simulink model "GridFormingConverter"  (R2025b)
settings: Solver=FixedStepAuto  StartTime=0.0  StopTime=simulationTime  FixedStep=gridInverter.vsm.samplingTime  MaxStep=gridInverter.vsm.samplingTime  RelTol=1e-3  AbsTol=1e-3
PreLoadFcn:
  | % Parameterize the model
  | GridFormingConverterInputParameters;
PostLoadFcn:
  | GridFormingConverterTestCondition;
undefined symbols (not defined in the file): base, DiscIntNeverNeededParam, Down, grid, gridInverter, k_smc1, k_smc2, L_smc, localSolverSampleTime, R_idsmc, scrFactorRg, scrFactorXg, transformer, TransmissionLine, Up
libraries: ee_lib x17, nesl_utility x17, eeGeneralControl x16, simulink x5, fl_lib x4, eeTransforms x4, eeSinGeneratorThreePhase x1, simulink_extras x1, eePowerMeasurement x1, eePwmGenerator x1
(part 2 of 3)

== system GridFormingConverter/Grid-Forming Converter/Grid-Forming Converter Control ==
  PrefPU : Inport
  QrefPU : Inport  Port=2
  IgabcPU : Inport  Port=3
  VgabcPU : Inport  Port=4
  Current Limiting : Subsystem
  Grid Voltage Reactive Power Support : Subsystem
  Measurement : Subsystem
      mask Display: image('$imagefile'); % Use "Edit Image" on toolstrip to change.
  Power Control : Subsystem
  Rate Transition3 : RateTransition
  VoltageCurrentControl : Subsystem
      settings: PortSchema="{\"entries\":[{\"content\":{\"sides\":[{\"content\":{\"connectorIds\":[\"In1\",\"In2\"]},\"type\":\"ConnectorPlacement.EquallySpacedRectSide\",\"uuid\":\"0bf15a12-7bc0-47e4-89bd-435769673763\"},{\"content\":{\"connectorIds\":[\"Out1\"],\"side\":\"RIGHT\"},\"type\":\"ConnectorPlacement.EquallySpacedRectSide\",\"uuid\":\"44a15d74-8878-4ec6-abe4-be0b1b609519\"},{\"content\":{\"connectorIds\":[\"In3\"],\"side\":\"TOP\"},\"type\":\"ConnectorPlacement.EquallySpacedRectSide\",\"uuid\":\"7a96781e-5638-4b2a-8101-d5785aae9f0f\"}]},\"type\":\"ConnectorPlacement.EquallySpacedConnector\",\"uuid\":\"4b3373ad-cf20-4175-894e-3bd1604dd0ce\"}],\"packageUris\":[\"http://schema.mathworks.com/mf0/Connector/R2020b\"],\"version\":\"1.0\"}"
  PmeasPU : Outport
  QmeasPU : Outport  Port=2
  FmeasHz : Outport  Port=3
  mabc : Outport  Port=4
  wires:
  VoltageCurrentControl/1(mabc) -> mabc/1
  VgabcPU/1 -> Measurement/1(Vgabcc)
  IgabcPU/1 -> Measurement/2(Igabc)
  Measurement/2(PmeasPU) -> PmeasPU/1
  Measurement/3(QmeasPU) -> QmeasPU/1
  Measurement/1(measure) -> Rate Transition3/1
  Power Control/3(angle) -> Measurement/3(Angle)
  Power Control/1(reactiveControl) -> Current Limiting/2(reactiveControl)
  Current Limiting/1(currentLimiting) -> VoltageCurrentControl/1(currentLimiting)
  QrefPU/1 -> Grid Voltage Reactive Power Support/3(QrefInput)
  PrefPU/1 -> Grid Voltage Reactive Power Support/2(PrefInput)
  Grid Voltage Reactive Power Support/1(Pref) -> Power Control/2(Pref)
  Grid Voltage Reactive Power Support/2(Qref) -> Power Control/3(Qref)
  Measurement/4(FmeasHz) -> FmeasHz/1
  Rate Transition3/1 -> Current Limiting/1(measure), VoltageCurrentControl/3(measure), Power Control/1(measure), Grid Voltage Reactive Power Support/1(measure)
  Power Control/2(activeControl) -> VoltageCurrentControl/2(activeControl)

== system GridFormingConverter/Grid-Forming Converter/Grid-Forming Converter Power Circuit ==
  mabc : Inport
  Average-Value : Subsystem  VariantControl=Average
  Switching : Subsystem  VariantControl=Switching
  P : PMIOPort  Side=Left
  N : PMIOPort  Port=2  Side=Left
  ABC : PMIOPort  Port=3  Side=Right

== system GridFormingConverter/Grid-Forming Converter/Grid-Forming Converter Control/Current Limiting ==
  In Bus Element : Inport  PortName=measure  Element=Igd
  In Bus Element1 : Inport  PortName=measure  Element=Igq
  In Bus Element2 : Inport  Port=2  PortName=reactiveControl  Element=Vmd
  In Bus Element4 : Inport  Port=2  PortName=reactiveControl  Element=Vmq
  CurrentLimitingMethod : Subsystem  Variant=on  VariantControlMode=label  VariantControl=Choice  LabelModeActiveChoice=virimp
  Subtract : Sum  Inputs=+-
  Subtract1 : Sum  Inputs=-+
  Out Bus Element : Outport  PortName=currentLimiting  Element=Vmd
  Out Bus Element1 : Outport  PortName=currentLimiting  Element=Vmq
  Out Bus Element2 : Outport  PortName=currentLimiting  Element=Idmax
  Out Bus Element3 : Outport  PortName=currentLimiting  Element=Iqmax
  wires:
  In Bus Element2/1 -> Subtract/1
  In Bus Element1/1 -> CurrentLimitingMethod/2(Igq)
  In Bus Element4/1 -> Subtract1/2
  Subtract/1 -> Out Bus Element/1
  Subtract1/1 -> Out Bus Element1/1
  In Bus Element/1 -> CurrentLimitingMethod/1(Igd)  "Q"
  CurrentLimitingMethod/1(delVd) -> Subtract/2
  CurrentLimitingMethod/2(delVq) -> Subtract1/1
  CurrentLimitingMethod/3(Idmax) -> Out Bus Element2/1
  CurrentLimitingMethod/4(Iqmax) -> Out Bus Element3/1

== system GridFormingConverter/Grid-Forming Converter/Grid-Forming Converter Control/Grid Voltage Reactive Power Support ==
  In Bus Element1 : Inport  PortName=measure  Element=Vgd
  In Bus Element3 : Inport  PortName=measure  Element=Vgq
  In Bus Element2 : Inport  PortName=measure  Element=Igd
  In Bus Element4 : Inport  PortName=measure  Element=Igq
  PrefInput : Inport  Port=2
  QrefInput : Inport  Port=3
  Modifying Active Power Reference : Subsystem
  Modifying Reactive Power Reference : Subsystem
  Rate Transition{,1..5} (6 alike) : RateTransition
  Pref : Outport
  Qref : Outport  Port=2
  wires:
  PrefInput/1 -> Modifying Active Power Reference/1(PrefInput)
  In Bus Element2/1 -> Modifying Active Power Reference/3(Igd)
  In Bus Element4/1 -> Modifying Active Power Reference/4(Igq)
  In Bus Element3/1 -> Rate Transition2/1
  QrefInput/1 -> Rate Transition3/1
  Modifying Reactive Power Reference/1(PrefNew) -> Rate Transition4/1
  Modifying Reactive Power Reference/2(QrefNew) -> Rate Transition5/1
  In Bus Element1/1 -> Rate Transition/1
  Modifying Active Power Reference/1(Pref) -> Rate Transition1/1
  Rate Transition2/1 -> Modifying Reactive Power Reference/2(Vgq)
  Rate Transition3/1 -> Modifying Reactive Power Reference/3(Qref)
  Rate Transition1/1 -> Modifying Reactive Power Reference/4(Pref)
  Rate Transition4/1 -> Pref/1
  Rate Transition5/1 -> Qref/1
  Rate Transition/1 -> Modifying Reactive Power Reference/1(Vgd), Modifying Active Power Reference/2(Vd)

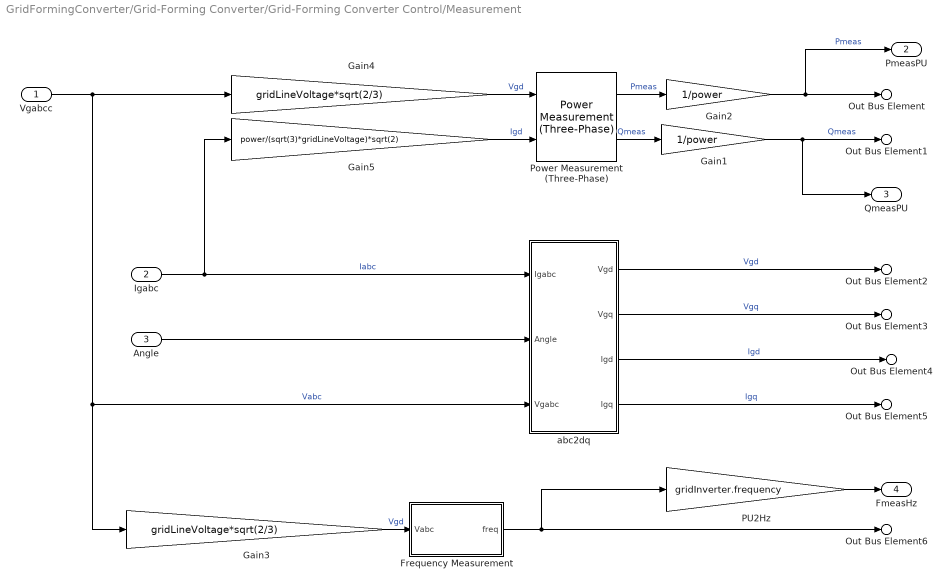
== system GridFormingConverter/Grid-Forming Converter/Grid-Forming Converter Control/Measurement ==
  Vgabcc : Inport
  Igabc : Inport  Port=2
  Angle : Inport  Port=3
  Frequency Measurement : Subsystem
  Gain1 : Gain  Gain=1/power
  Gain2 : Gain  Gain=1/power
  Gain3 : Gain  Gain=gridLineVoltage*sqrt(2/3)
  Gain4 : Gain  Gain=gridLineVoltage*sqrt(2/3)
  Gain5 : Gain  Gain=power/(sqrt(3)*gridLineVoltage)*sqrt(2)
  PU2Hz : Gain  Gain=gridInverter.frequency
  Power Measurement (Three-Phase) : eePowerMeasurement/Power Measurement (Three-Phase)  LabelModeActiveChoice=Discrete  F=powerFreq  K=[1]  Seq=Positive  Ts=measSampleTime
  abc2dq : Subsystem
  Out Bus Element : Outport  PortName=measure  Element=P
  Out Bus Element1 : Outport  PortName=measure  Element=Q
  Out Bus Element2 : Outport  PortName=measure  Element=Vgd
  Out Bus Element3 : Outport  PortName=measure  Element=Vgq
  Out Bus Element4 : Outport  PortName=measure  Element=Igd
  Out Bus Element5 : Outport  PortName=measure  Element=Igq
  Out Bus Element6 : Outport  PortName=measure  Element=fgrid
  PmeasPU : Outport  Port=2
  QmeasPU : Outport  Port=3
  FmeasHz : Outport  Port=4
  wires:
  Vgabcc/1 -> abc2dq/3(Vgabc), Gain3/1, Gain4/1  "Vabc"
  Angle/1 -> abc2dq/2(Angle)
  Igabc/1 -> Gain5/1, abc2dq/1(Igabc)  "Iabc"
  abc2dq/2(Vgq) -> Out Bus Element3/1  "Vgq"
  abc2dq/1(Vgd) -> Out Bus Element2/1  "Vgd"
  abc2dq/3(Igd) -> Out Bus Element4/1  "Igd"
  abc2dq/4(Igq) -> Out Bus Element5/1  "Igq"
  Frequency Measurement/1(freq) -> PU2Hz/1, Out Bus Element6/1
  PU2Hz/1 -> FmeasHz/1
  Power Measurement (Three-Phase)/1 -> Gain2/1  "Pmeas"
  Power Measurement (Three-Phase)/2 -> Gain1/1  "Qmeas"
  Gain4/1 -> Power Measurement (Three-Phase)/1  "Vgd"
  Gain5/1 -> Power Measurement (Three-Phase)/2  "Igd"
  Gain2/1 -> Out Bus Element/1, PmeasPU/1  "Pmeas"
  Gain1/1 -> QmeasPU/1, Out Bus Element1/1  "Qmeas"
  Gain3/1 -> Frequency Measurement/1(Vabc)  "Vgd"

== system GridFormingConverter/Grid-Forming Converter/Grid-Forming Converter Control/Power Control ==
  note: Reactive Power Control
  note: Active Power Control
  In Bus Element2 : Inport  PortName=measure  Element=P
  In Bus Element3 : Inport  PortName=measure  Element=Q
  In Bus Element1 : Inport  PortName=measure  Element=fgrid
  Pref : Inport  Port=2
  Qref : Inport  Port=3
  ActivePowerControl : Subsystem  Variant=on  VariantControlMode=label  VariantControl=Choice  LabelModeActiveChoice=vsm
  ReactiveControl : Subsystem
  Out Bus Element : Outport  PortName=reactiveControl  Element=Vmd
  Out Bus Element1 : Outport  PortName=reactiveControl  Element=Vmq
  Out Bus Element6 : Outport  Port=2  PortName=activeControl  Element=angle
  Out Bus Element4 : Outport  Port=2  PortName=activeControl  Element=w
  angle : Outport  Port=3
  wires:
  ActivePowerControl/2(w) -> Out Bus Element4/1
  In Bus Element3/1 -> ReactiveControl/2(Qmeas)
  ActivePowerControl/1(Theta) -> angle/1, Out Bus Element6/1
  ReactiveControl/1(Vmd) -> Out Bus Element/1
  ReactiveControl/2(Vmq) -> Out Bus Element1/1
  Pref/1 -> ActivePowerControl/1(Pref)  "Q"
  Qref/1 -> ReactiveControl/1(Qref)  "Q"
  In Bus Element2/1 -> ActivePowerControl/2(Pmeas)
  In Bus Element1/1 -> ActivePowerControl/3(fgrid)

== system GridFormingConverter/Grid-Forming Converter/Grid-Forming Converter Control/VoltageCurrentControl ==
  In Bus Element : Inport  PortName=currentLimiting  Element=Vmd
  In Bus Element1 : Inport  PortName=currentLimiting  Element=Vmq
  In Bus Element6 : Inport  PortName=currentLimiting  Element=Idmax
  In Bus Element7 : Inport  PortName=currentLimiting  Element=Iqmax
  Bus Element In6 : Inport  Port=2  PortName=activeControl  Element=w
  Bus Element In1 : Inport  Port=2  PortName=activeControl  Element=angle
  In Bus Element2 : Inport  Port=3  PortName=measure  Element=Vgd
  In Bus Element3 : Inport  Port=3  PortName=measure  Element=Vgq
  In Bus Element4 : Inport  Port=3  PortName=measure  Element=Igd
  In Bus Element5 : Inport  Port=3  PortName=measure  Element=Igq
  Controller : Subsystem
  Modulation Signal : Subsystem
  mabc : Outport
  wires:
  Controller/2(Vq) -> Modulation Signal/2(Vq)
  Modulation Signal/1(mabc) -> mabc/1
  Controller/1(Vd) -> Modulation Signal/1(Vd)
  In Bus Element4/1 -> Controller/6(Id)
  In Bus Element5/1 -> Controller/7(Iq)
  In Bus Element6/1 -> Controller/8(Idmax)
  In Bus Element7/1 -> Controller/9(Iqmax)
  In Bus Element2/1 -> Controller/4(Vsd)
  In Bus Element3/1 -> Controller/5(Vsq)
  Bus Element In6/1 -> Controller/1(Angfreq)
  In Bus Element/1 -> Controller/2(Vgdref)
  In Bus Element1/1 -> Controller/3(Vgqref)
  Bus Element In1/1 -> Modulation Signal/3(Angle)

== system GridFormingConverter/Grid-Forming Converter/Grid-Forming Converter Power Circuit/Average-Value ==
  mabc : Inport
  Electrical Reference : fl_lib/Electrical/Electrical Elements/Electrical Reference
  Grid Forming Converter : ee_lib/Semiconductors & Converters/Converters/Average-Value Voltage Source Converter (Three-Phase)  port_option=ee.enum.threePhasePort.composite  frequency_option=ee.enum.converters.frequency.variable  input_option=ee.enum.converters.inputOption.ModWave  FRated=50 Hz  losses_parameterization=ee.enum.converters.losses.fixed  Pfixed=10 W  ks=0.01  kc1=1.7 V  kc2=0.01 Ohm  Ploss_vect=[100, 800, 1870, 3250, 4900] W  Irms_vect=[10, 100, 200, 300, 400] A  Vdc_nom=300 V  thermal_mass=30000 J/K  temperature_specify=off  temperature_priority=High  temperature=298.15 K  temperature_nominal_specify=off  temperature_nominal_value=1  temperature_nominal_unit=K
      settings: InternalSimscapePortConfiguration="{\"Bottom\":[],\"Left\":[{\"id\":\"ModWave\",\"label\":\"ModWave\",\"type\":\"input\"},{\"id\":\"N\",\"label\":\"~\",\"type\":\"foundation.electrical.three_phase\"}],\"Right\":[{\"id\":\"p\",\"label\":\"+\",\"type\":\"foundation.electrical.electrical\"},{\"id\":\"n\",\"label\":\"-\",\"type\":\"foundation.electrical.electrical\"}],\"Top\":[]}"
  Simulink-PS Converter : nesl_utility/Simulink-PS Converter  PhysicalDomain=network_engine_domain  SubClassName=ps_input  LeftPortType=input  RightPortType=output  PseudoPeriodic=off  Frequencies=[]  NoiseDistribution=none  NoiseParameters=[]  Unit=1  AffineConversion=off  FilteringAndDerivatives=provide  SimscapeFilterOrder=1  InputFilterTimeConstant=0.001  UdotUserProvided=0
  P : PMIOPort  Side=Left
  N : PMIOPort  Port=2  Side=Left
  ABC : PMIOPort  Port=3  Side=Right
  wires:
  mabc/1 -> Simulink-PS Converter/1
  connections:
  ABC/RConn1 -- Grid Forming Converter/LConn2
  Simulink-PS Converter/RConn1 -- Grid Forming Converter/LConn1
  P/RConn1 -- Grid Forming Converter/RConn1
  Grid Forming Converter/RConn2 -- Electrical Reference/LConn1 -- N/RConn1

== system GridFormingConverter/Grid-Forming Converter/Grid-Forming Converter Power Circuit/Switching ==
  mabc : Inport
  Converter (Three-Phase) : ee_lib/Semiconductors & Converters/Converters/Converter (Three-Phase)  port_option=ee.enum.threePhasePort.composite  fidelity_option=ee.enum.converters.fidelity.detailed  device_type=ee.enum.converters.switchingdevice.ideal  showThermalPort=false  K=0  Vth=0.5 V  Vgt=1 V  Vgt_off=-1 V  Ih=1 A  Vf=0.8 V  Ron=0.001 Ohm  Rds=0.001 Ohm  Goff=1e-6 1/Ohm  Eon_scalar=22.86e-3 J  Eoff_scalar=17.14e-3 J  Eoff_natural_commutation=10e-3 J  Voff=300 V  Iout_scalar=600 A  onCurrentMeasDelay=0 s  useCurrentFromPreviousCycle=false  useVoltageFromPreviousCycle=false  diode_param=ee.enum.converters.protectiondiode.nodynamics  diode_Vf=0.01 V  diode_Ron=0.0001 Ohm  diode_Goff=1e-5 1/Ohm  diode_C=50 nF  diode_iRM=-235 A  diode_iF=300 A  diode_idot=-50 A/us  diode_trr_param=ee.enum.converters.diodetrr.trr_factor  diode_trr_factor=3  diode_trr=15 us  diode_Qrr=1500 s*uA  diode_rec_loss_model=ee.enum.diode.reverseRecoveryModel.fixed  diode_ErecVal=0 J  diode_scaleWithIandV=false  diode_ErecMat=zeros(2, 3) J  diode_TjrecVec=[298.15, 398.15] K  diode_IfrecVec=[.1, 1, 10] A  diode_IrecVal=10 A  diode_VrecVal=10 V  diode_tFilter=1 / 1000 / 100 s  thermal_network_parameterization=ee.enum.thermalNetworkTopology.external  Rth=[.08, .5] K/W  Rth_Cauer=[.08, .1, .5] K/W  Rth_Foster=[.08, .14, .22, .16] K/W  thermal_mass_parameterization=ee.enum.thermalNetwork.timeconstant  thermal_mass=[.01, .5] J/K  thermal_mass_Cauer=[.01, .1, .5] J/K  thermal_mass_Foster=[.001, .005, .05, .5] J/K  thermal_time_constant=[.001, .2] s  thermal_time_constant_Cauer=[.001, .1, .2] s  thermal_time_constant_Foster=[7e-05, .0007, .01, .08] s  thermal_mass_initial_temperatures=[25, 25] degC  thermal_mass_initial_temperatures_Cauer=[25, 25, 25] degC  junction_thermal_mass=0.01 J/K  Tvec_initial_Foster=[25, 25, 25, 25] degC  snubber_type=ee.enum.converters.snubber.exclude  Cs=1e-7 F  Rs=0.1 Ohm  Vce_loss=[0, 150, 300] V
  Mod2PWM SIgnal : Subsystem
  Simulink-PS Converter{1..6} (6 alike) : nesl_utility/Simulink-PS Converter  PhysicalDomain=network_engine_domain  SubClassName=ps_input  LeftPortType=input  RightPortType=output  PseudoPeriodic=off  Frequencies=[]  NoiseDistribution=none  NoiseParameters=[]  Unit=1  AffineConversion=off  FilteringAndDerivatives=provide  SimscapeFilterOrder=1  InputFilterTimeConstant=0.001  UdotUserProvided=0
  Six-Pulse Gate Multiplexer : ee_lib/Semiconductors & Converters/Converters/Six-Pulse Gate Multiplexer  port_option=ee.enum.controlport.ps
  P : PMIOPort  Side=Left
  N : PMIOPort  Port=2  Side=Left
  ABC : PMIOPort  Port=3  Side=Right
  wires:
  mabc/1 -> Mod2PWM SIgnal/1(mod)
  Mod2PWM SIgnal/1(AH) -> Simulink-PS Converter6/1
  Mod2PWM SIgnal/2(AL) -> Simulink-PS Converter5/1
  Mod2PWM SIgnal/3(BH) -> Simulink-PS Converter4/1
  Mod2PWM SIgnal/4(BL) -> Simulink-PS Converter3/1
  Mod2PWM SIgnal/5(CH) -> Simulink-PS Converter2/1
  Mod2PWM SIgnal/6(CL) -> Simulink-PS Converter1/1
  connections:
  Six-Pulse Gate Multiplexer/RConn1 -- Converter (Three-Phase)/LConn1
  P/RConn1 -- Converter (Three-Phase)/RConn1
  Six-Pulse Gate Multiplexer/LConn2 -- Simulink-PS Converter5/RConn1
  Simulink-PS Converter2/RConn1 -- Six-Pulse Gate Multiplexer/LConn5
  Simulink-PS Converter1/RConn1 -- Six-Pulse Gate Multiplexer/LConn6
  Six-Pulse Gate Multiplexer/LConn1 -- Simulink-PS Converter6/RConn1
  N/RConn1 -- Converter (Three-Phase)/RConn2
  Six-Pulse Gate Multiplexer/LConn3 -- Simulink-PS Converter4/RConn1
  Six-Pulse Gate Multiplexer/LConn4 -- Simulink-PS Converter3/RConn1
  Converter (Three-Phase)/LConn2 -- ABC/RConn1

== system GridFormingConverter/Grid-Forming Converter/Grid-Forming Converter Control/Current Limiting/CurrentLimitingMethod ==
  Igd : Inport
  Igq : Inport  Port=2
  currentLimitAndVirtual : Subsystem  VariantControl=both
  currentSaturation : Subsystem  VariantControl=ctSat
  virtualImpedance : Subsystem  VariantControl=virimp
  delVd : Outport
  delVq : Outport  Port=2
  Idmax : Outport  Port=3
  Iqmax : Outport  Port=4

== system GridFormingConverter/Grid-Forming Converter/Grid-Forming Converter Control/Grid Voltage Reactive Power Support/Modifying Active Power Reference ==
  PrefInput : Inport
  Vd : Inport  Port=2
  Igd : Inport  Port=3
  Igq : Inport  Port=4
  AND : Logic  IconShape=distinctive  AllPortsSameDT=off  OutDataTypeStr=boolean
  Abs : Abs  SaturateOnIntegerOverflow=off
  Compare To Constant : simulink/Logic and Bit Operations/Compare To Constant  relop=<=  const=0.90  OutDataTypeStr=boolean
  Computing New Active Power Ref : Subsystem
  Math Function1 : Math  Operator=hypot
  Power Sign : Signum
  Product : Product
  Rate Transition1 : RateTransition
  Relay : Relay  OnSwitchValue=maxVICurrentLimit*0.96  OffSwitchValue=1
  Switch : Switch  Criteria=u2 > Threshold  SaturateOnIntegerOverflow=off  InputSameDT=off
  Pref : Outport
  wires:
  Computing New Active Power Ref/1(Pref) -> Switch/1
  Math Function1/1 -> Rate Transition1/1  "Is"
  Vd/1 -> Computing New Active Power Ref/2(Vd), Compare To Constant/1
  PrefInput/1 -> Power Sign/1, Switch/3
  Igd/1 -> Math Function1/2
  Switch/1 -> Abs/1
  Abs/1 -> Product/1
  Power Sign/1 -> Product/2
  Product/1 -> Pref/1
  Relay/1 -> AND/2
  AND/1 -> Switch/2
  Compare To Constant/1 -> AND/1
  Igq/1 -> Computing New Active Power Ref/1(Iq), Math Function1/1
  Rate Transition1/1 -> Relay/1

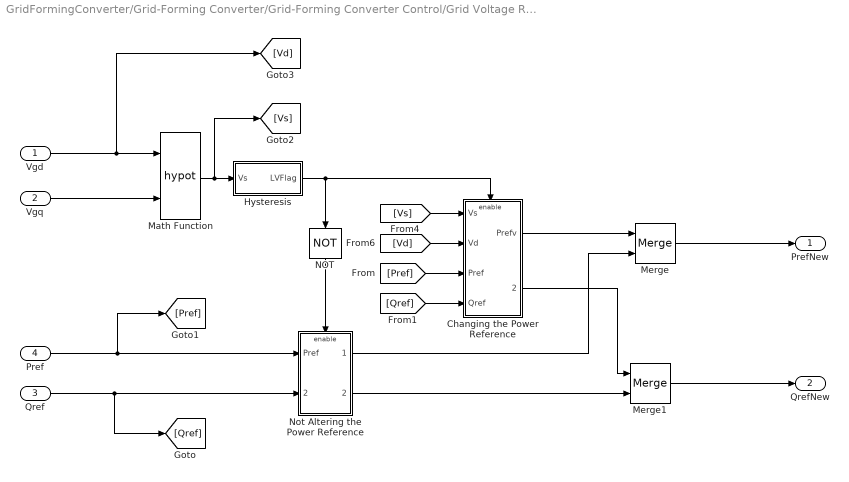
== system GridFormingConverter/Grid-Forming Converter/Grid-Forming Converter Control/Grid Voltage Reactive Power Support/Modifying Reactive Power Reference ==
  Vgd : Inport
  Vgq : Inport  Port=2
  Qref : Inport  Port=3
  Pref : Inport  Port=4
  Changing the Power Reference : Subsystem
  Hysteresis : Subsystem
  Math Function : Math  Operator=hypot
  Merge : Merge
  Merge1 : Merge
  NOT : Logic  Operator=NOT  IconShape=distinctive  AllPortsSameDT=off  OutDataTypeStr=boolean
  Not Altering the Power Reference : Subsystem
  PrefNew : Outport
  QrefNew : Outport  Port=2
  wires:
  Vgd/1 -> [Vd], Math Function/1
  Not Altering the Power Reference/2(Qrefv) -> Merge1/2
  Math Function/1 -> Hysteresis/1(Vs), [Vs]
  [Vs] -> Changing the Power Reference/1(Vs)
  Not Altering the Power Reference/1(Prefv) -> Merge/2
  Changing the Power Reference/1(Prefv) -> Merge/1
  NOT/1 -> Not Altering the Power Reference/Enable
  Qref/1 -> Not Altering the Power Reference/2(Qref), [Qref]
  Hysteresis/1(LVFlag) -> Changing the Power Reference/Enable, NOT/1
  [Vd] -> Changing the Power Reference/2(Vd)
  Changing the Power Reference/2(Qrefv) -> Merge1/1
  Vgq/1 -> Math Function/2
  Pref/1 -> Not Altering the Power Reference/1(Pref), [Pref]
  Merge1/1 -> QrefNew/1
  Merge/1 -> PrefNew/1
  [Pref] -> Changing the Power Reference/3(Pref)
  [Qref] -> Changing the Power Reference/4(Qref)

== system GridFormingConverter/Grid-Forming Converter/Grid-Forming Converter Control/Measurement/Frequency Measurement ==
  Vabc : Inport
  Convert To PU : Gain  Gain=1/powerFreq
  Frequency Measurement : Subsystem  TreatAsAtomicUnit=on  SystemSampleTime=sampleTime  mask{initialFrequency=powerFreq, sampleTime=activePowerSampleTime}
      mask prompts: initialFrequency "Initial frequency in Hz"; sampleTime "Sample time in sec"
      mask DialogControl Container7 Prompt: General
  Low-Pass Filter : eeGeneralControl/Low-Pass Filter (Discrete or Continuous)  K=1  T=freqMeasTimeConst  B=inf  A=-inf  init_option=Inherited from block input  x0=0  Ts=-1
  Low-Pass Filter1 : eeGeneralControl/Low-Pass Filter (Discrete or Continuous)  K=1  T=0.1/powerFreq  B=inf  A=-inf  init_option=Inherited from block input  x0=0  Ts=-1
  Saturation : Saturate  UpperLimit=1.1  LowerLimit=0.9
  freq : Outport
  wires:
  Low-Pass Filter/1 -> Convert To PU/1  "Freq"
  Frequency Measurement/1(Freq) -> Low-Pass Filter/1
  Convert To PU/1 -> Saturation/1
  Vabc/1 -> Low-Pass Filter1/1
  Low-Pass Filter1/1 -> Frequency Measurement/1(abc)
  Saturation/1 -> freq/1

== system GridFormingConverter/Grid-Forming Converter/Grid-Forming Converter Control/Measurement/abc2dq ==
  Igabc : Inport
  Angle : Inport  Port=2
  Vgabc : Inport  Port=3
  Supply Current to dq : Subsystem
  Supply Voltage  to dq : Subsystem
  Vgd : Outport
  Vgq : Outport  Port=2
  Igd : Outport  Port=3
  Igq : Outport  Port=4
  wires:
  Angle/1 -> Supply Voltage  to dq/1(Angle), Supply Current to dq/2(Angle)
  Vgabc/1 -> Supply Voltage  to dq/2(abc)
  Igabc/1 -> Supply Current to dq/1(abc)
  Supply Current to dq/1(Igd) -> Igd/1  "Id"
  Supply Current to dq/2(Igq) -> Igq/1  "Iq"
  Supply Voltage  to dq/1(Vgd) -> Vgd/1  "Vgd"
  Supply Voltage  to dq/2(Vgq) -> Vgq/1  "Vgq"

== system GridFormingConverter/Grid-Forming Converter/Grid-Forming Converter Control/Power Control/ActivePowerControl ==
  Pref : Inport
  Pmeas : Inport  Port=2
  fgrid : Inport  Port=3
  droopControl : Subsystem  VariantControl=droop
  vsmControl : Subsystem  VariantControl=vsm
  Theta : Outport
  w : Outport  Port=2

== system GridFormingConverter/Grid-Forming Converter/Grid-Forming Converter Control/Power Control/ReactiveControl ==
  note: Vs-delV
  Qref : Inport
  Qmeas : Inport  Port=2
  Constant : Constant  Value=voltreference
  Constant2 : Constant  Value=0
  Gain : Gain  Gain=QVoltDroop
  Low-Pass Filter (Discrete or Continuous) : eeGeneralControl/Low-Pass Filter (Discrete or Continuous)  K=1  T=QVoltFilterTC  B=inf  A=-inf  init_option=Specify as parameter  x0=0  Ts=activePowerSampleTime
  Product1 : Product
  Saturation1 : Saturate  UpperLimit=(dcBusVoltage/2)/(sqrt(2/3)*gridLineVoltage)  LowerLimit=-(dcBusVoltage/2)/(sqrt(2/3)*gridLineVoltage)
  Sum : Sum  Inputs=|+-
  Sum1 : Sum  Inputs=|++
  Vmd : Outport
  Vmq : Outport  Port=2
  wires:
  Sum/1 -> Gain/1
  Qmeas/1 -> Low-Pass Filter (Discrete or Continuous)/1
  Low-Pass Filter (Discrete or Continuous)/1 -> Sum/2
  Gain/1 -> Sum1/1
  Product1/1 -> Saturation1/1  "Q"
  Constant/1 -> Product1/2, Sum1/2
  Constant2/1 -> Vmq/1
  Sum1/1 -> Product1/1
  Qref/1 -> Sum/1
  Saturation1/1 -> Vmd/1

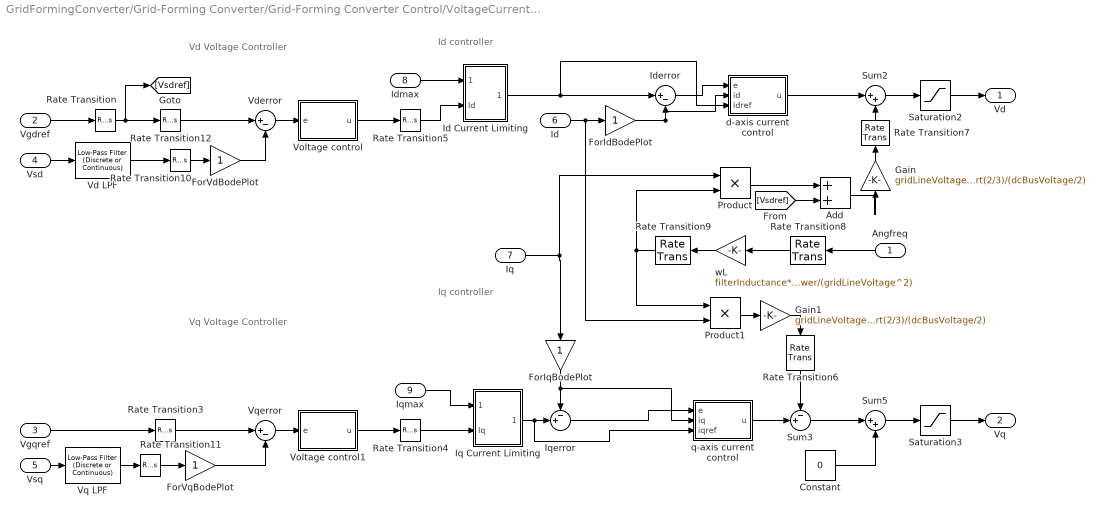
== system GridFormingConverter/Grid-Forming Converter/Grid-Forming Converter Control/VoltageCurrentControl/Controller ==
  note: Id controller
  note: Vd Voltage Controller
  note: Iq controller
  note: Vq Voltage Controller
  Angfreq : Inport
  Vgdref : Inport  Port=2
  Vgqref : Inport  Port=3
  Vsd : Inport  Port=4
  Vsq : Inport  Port=5
  Id : Inport  Port=6
  Iq : Inport  Port=7
  Idmax : Inport  Port=8
  Iqmax : Inport  Port=9
  Add : Sum
  Constant : Constant  Value=0  SampleTime=currentControlTs
  ForIdBodePlot : Gain
  ForIqBodePlot : Gain
  ForVdBodePlot : Gain
  ForVqBodePlot : Gain
  Gain : Gain  Gain=gridLineVoltage*sqrt(2/3)/(dcBusVoltage/2)
  Gain1 : Gain  Gain=gridLineVoltage*sqrt(2/3)/(dcBusVoltage/2)
  Id Current Limiting : Subsystem
  Iderror : Sum  Inputs=|+-
  Iq Current Limiting : Subsystem
  Iqerror : Sum  Inputs=-+|
  Product : Product
  Product1 : Product
  Rate Transition{,3..12} (11 alike) : RateTransition
  Saturation2 : Saturate  UpperLimit=4  LowerLimit=-3
  Saturation3 : Saturate  UpperLimit=3  LowerLimit=-3
  Sum2 : Sum  Inputs=|++
  Sum3 : Sum  Inputs=-+|
  Sum5 : Sum  Inputs=|++
  Vd LPF : eeGeneralControl/Low-Pass Filter (Discrete or Continuous)  K=1  T=vdvqLPFTimeConst  B=inf  A=-inf  init_option=Specify as parameter  x0=0  Ts=voltControlTs
  Vderror : Sum  Inputs=|+-
  Voltage control : Subsystem
  Voltage control1 : Subsystem
  Vq LPF : eeGeneralControl/Low-Pass Filter (Discrete or Continuous)  K=1  T=vdvqLPFTimeConst  B=inf  A=-inf  init_option=Inherited from block input  x0=0  Ts=voltControlTs
  Vqerror : Sum  Inputs=|+-
  d-axis current control : Subsystem
  q-axis current control : Subsystem
  wL : Gain  Gain=filterInductance*power/(gridLineVoltage^2)
  Vd : Outport  VectorParamsAs1DForOutWhenUnconnected=off
  Vq : Outport  Port=2  VectorParamsAs1DForOutWhenUnconnected=off
  wires:
  Iqerror/1 -> q-axis current control/1(e)
  wL/1 -> Rate Transition9/1
  Iq/1 -> ForIqBodePlot/1, Product/1
  Angfreq/1 -> Rate Transition8/1
  Constant/1 -> Sum5/2
  Iderror/1 -> d-axis current control/1(e)
  Saturation3/1 -> Vq/1
  Saturation2/1 -> Vd/1
  Product1/1 -> Gain1/1
  Product/1 -> Add/1
  d-axis current control/1(u) -> Sum2/1
  q-axis current control/1(u) -> Sum3/2
  Sum3/1 -> Sum5/1
  Vsq/1 -> Vq LPF/1
  Id/1 -> Product1/2, ForIdBodePlot/1
  Vderror/1 -> Voltage control/1(e)
  Iqmax/1 -> Iq Current Limiting/1(Imax)
  Vgqref/1 -> Rate Transition3/1
  Vqerror/1 -> Voltage control1/1(e)
  Gain1/1 -> Rate Transition6/1
  [Vsdref] -> Add/2
  Add/1 -> Gain/1
  Gain/1 -> Rate Transition7/1
  Voltage control/1(u) -> Rate Transition5/1
  Idmax/1 -> Id Current Limiting/1(Imax)
  Iq Current Limiting/1(Iqref) -> q-axis current control/3(iqref), Iqerror/2
  Voltage control1/1(u) -> Rate Transition4/1
  Vsd/1 -> Vd LPF/1
  ForIdBodePlot/1 -> d-axis current control/2(id), Iderror/2
  ForIqBodePlot/1 -> q-axis current control/2(iq), Iqerror/1
  Id Current Limiting/1(Idref) -> d-axis current control/3(idref), Iderror/1
  Vgdref/1 -> Rate Transition/1
  Rate Transition/1 -> [Vsdref], Rate Transition12/1
  Rate Transition3/1 -> Vqerror/1
  Rate Transition4/1 -> Iq Current Limiting/2(Iq)
  Rate Transition5/1 -> Id Current Limiting/2(Id)
  Rate Transition6/1 -> Sum3/1
  Rate Transition7/1 -> Sum2/2
  Rate Transition8/1 -> wL/1
  Vq LPF/1 -> Rate Transition11/1
  Rate Transition9/1 -> Product/2, Product1/1
  ForVdBodePlot/1 -> Vderror/2
  ForVqBodePlot/1 -> Vqerror/2
  Vd LPF/1 -> Rate Transition10/1
  Rate Transition10/1 -> ForVdBodePlot/1
  Rate Transition11/1 -> ForVqBodePlot/1
  Rate Transition12/1 -> Vderror/1
  Sum5/1 -> Saturation3/1
  Sum2/1 -> Saturation2/1

== system GridFormingConverter/Grid-Forming Converter/Grid-Forming Converter Control/VoltageCurrentControl/Modulation Signal ==
  Vd : Inport
  Vq : Inport  Port=2
  Angle : Inport  Port=3
  Constant : Constant  Value=0
  Inverse Park Transform : eeTransforms/Inverse Park Transform  AxisAlignment=D-axis  PowerInvariant=off
  Mux1 : Mux  Inputs=3
  Saturation2 : Saturate  UpperLimit=1  LowerLimit=-1
  mabc : Outport  VectorParamsAs1DForOutWhenUnconnected=off
  wires:
  Inverse Park Transform/1 -> Saturation2/1
  Mux1/1 -> Inverse Park Transform/1
  Saturation2/1 -> mabc/1
  Constant/1 -> Mux1/3
  Vd/1 -> Mux1/1
  Angle/1 -> Inverse Park Transform/2
  Vq/1 -> Mux1/2

== system GridFormingConverter/Grid-Forming Converter/Grid-Forming Converter Power Circuit/Switching/Mod2PWM SIgnal ==
  mod : Inport
  Add : Sum
  Constant : Constant
  Constant1 : Constant
  Demux : Demux  Outputs=3
  Demux1 : Demux  Outputs=3
  Gain : Gain
  Gain1 : Gain  Gain=0.5
  PWM Generator : eePwmGenerator/PWM Generator  CarrCount=Up-Down  Tper=1/gridInverter.switchingFrequency  Tdelay=0  Ts=1/(10*gridInverter.switchingFrequency)
  Rate Transition1 : RateTransition  OutPortSampleTime=1/(10*gridInverter.switchingFrequency)
  Subtract : Sum  Inputs=-+
  AH : Outport
  AL : Outport  Port=2
  BH : Outport  Port=3
  BL : Outport  Port=4
  CH : Outport  Port=5
  CL : Outport  Port=6
  wires:
  Gain/1 -> Demux/1, Subtract/1
  Gain1/1 -> Rate Transition1/1
  Constant1/1 -> Add/2
  PWM Generator/1 -> Gain/1
  mod/1 -> Add/1
  Add/1 -> Gain1/1
  Rate Transition1/1 -> PWM Generator/1
  Subtract/1 -> Demux1/1
  Constant/1 -> Subtract/2
  Demux1/2 -> BL/1
  Demux1/3 -> CL/1
  Demux/1 -> AH/1
  Demux1/1 -> AL/1
  Demux/2 -> BH/1
  Demux/3 -> CH/1

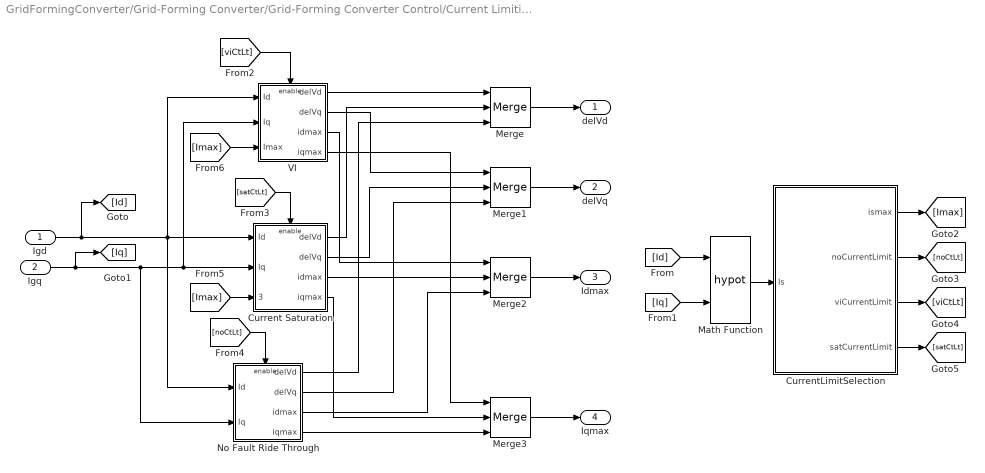
== system GridFormingConverter/Grid-Forming Converter/Grid-Forming Converter Control/Current Limiting/CurrentLimitingMethod/currentLimitAndVirtual ==
  Igd : Inport
  Igq : Inport  Port=2
  Current Saturation : Subsystem
  CurrentLimitSelection : Stateflow chart  TreatAsAtomicUnit=on
  Math Function : Math  Operator=hypot
  Merge{,1..3} (4 alike) : Merge  Inputs=3
  No Fault Ride Through : Subsystem
  VI : Subsystem
  delVd : Outport
  delVq : Outport  Port=2
  Idmax : Outport  Port=3
  Iqmax : Outport  Port=4
  wires:
  Merge2/1 -> Idmax/1
  Igq/1 -> Current Saturation/2(Iq), VI/2(Iq), No Fault Ride Through/2(Iq), [Iq]
  Merge1/1 -> delVq/1
  Igd/1 -> VI/1(Id), Current Saturation/1(Id), No Fault Ride Through/1(Id), [Id]
  No Fault Ride Through/1(delVd) -> Merge/3
  No Fault Ride Through/3(idmax) -> Merge2/3
  VI/1(delVd) -> Merge/1
  [Iq] -> Math Function/2
  [Id] -> Math Function/1
  Current Saturation/1(delVd) -> Merge/2
  Current Saturation/4(iqmax) -> Merge3/2
  Merge/1 -> delVd/1
  VI/2(delVq) -> Merge1/1
  Current Saturation/3(idmax) -> Merge2/2
  VI/4(iqmax) -> Merge3/1
  VI/3(idmax) -> Merge2/1
  No Fault Ride Through/4(iqmax) -> Merge3/3
  Current Saturation/2(delVq) -> Merge1/2
  Merge3/1 -> Iqmax/1
  No Fault Ride Through/2(delVq) -> Merge1/3
  Math Function/1 -> CurrentLimitSelection/1(Is)
  CurrentLimitSelection/1(ismax) -> [Imax]
  CurrentLimitSelection/2(noCurrentLimit) -> [noCtLt]
  CurrentLimitSelection/3(viCurrentLimit) -> [viCtLt]
  CurrentLimitSelection/4(satCurrentLimit) -> [satCtLt]
  [viCtLt] -> VI/Enable
  [satCtLt] -> Current Saturation/Enable
  [noCtLt] -> No Fault Ride Through/Enable
  [Imax] -> Current Saturation/3(Imaxsat)
  [Imax] -> VI/3(Imax)

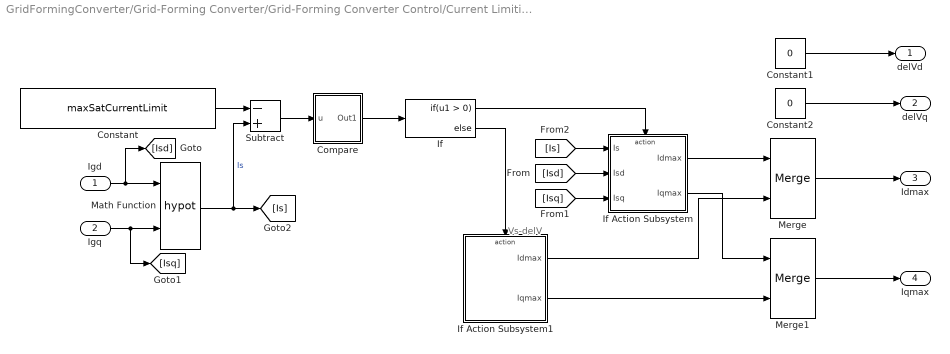
== system GridFormingConverter/Grid-Forming Converter/Grid-Forming Converter Control/Current Limiting/CurrentLimitingMethod/currentSaturation ==
  note: Vs-delV
  Igd : Inport
  Igq : Inport  Port=2
  Compare : Subsystem
  Constant : Constant  Value=maxSatCurrentLimit
  Constant1 : Constant  Value=0
  Constant2 : Constant  Value=0
  If : If
  If Action Subsystem : Subsystem  TreatAsAtomicUnit=on
  If Action Subsystem1 : Subsystem  TreatAsAtomicUnit=on
  Math Function : Math  Operator=hypot
  Merge : Merge
  Merge1 : Merge
  Subtract : Sum  Inputs=-+
  delVd : Outport
  delVq : Outport  Port=2
  Idmax : Outport  Port=3
  Iqmax : Outport  Port=4
  wires:
  Igd/1 -> [Isd], Math Function/1
  Igq/1 -> [Isq], Math Function/2
  Constant/1 -> Subtract/1
  Math Function/1 -> [Is], Subtract/2  "Is"
  If/1 -> If Action Subsystem/Action
  [Isd] -> If Action Subsystem/2(Isd)
  [Isq] -> If Action Subsystem/3(Isq)
  Subtract/1 -> Compare/1(u)
  Compare/1(Out1) -> If/1
  If/2 -> If Action Subsystem1/Action
  [Is] -> If Action Subsystem/1(Is)
  If Action Subsystem/1(Idmax) -> Merge/1
  If Action Subsystem1/1(Idmax) -> Merge/2
  If Action Subsystem/2(Iqmax) -> Merge1/1
  If Action Subsystem1/2(Iqmax) -> Merge1/2
  Constant2/1 -> delVq/1
  Constant1/1 -> delVd/1
  Merge/1 -> Idmax/1
  Merge1/1 -> Iqmax/1

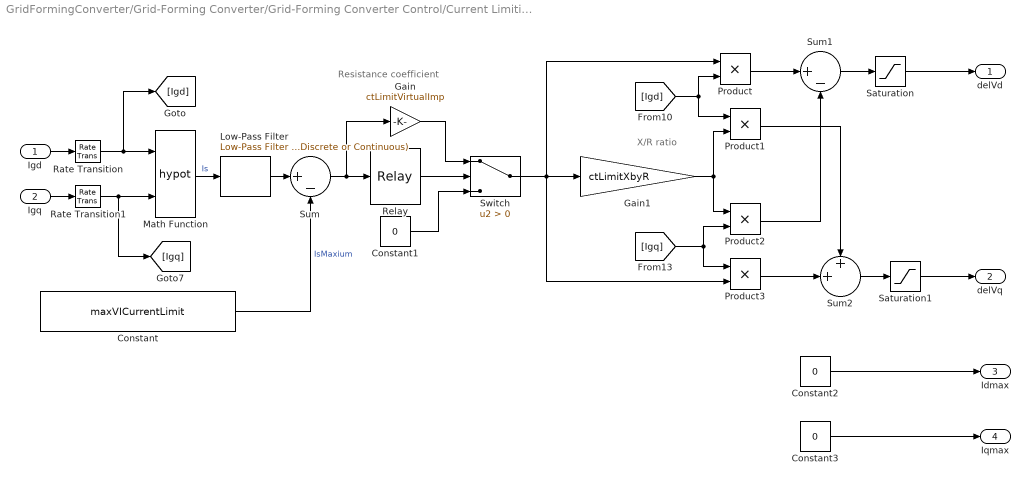
== system GridFormingConverter/Grid-Forming Converter/Grid-Forming Converter Control/Current Limiting/CurrentLimitingMethod/virtualImpedance ==
  note: X/R ratio
  note: Resistance coefficient
  Igd : Inport
  Igq : Inport  Port=2
  Constant : Constant  Value=maxVICurrentLimit
  Constant1 : Constant  Value=0
  Constant2 : Constant  Value=0
  Constant3 : Constant  Value=0
  Gain : Gain  Gain=ctLimitVirtualImp
  Gain1 : Gain  Gain=ctLimitXbyR
  Low-Pass Filter : eeGeneralControl/Low-Pass Filter (Discrete or Continuous)  K=1  T=currentVITimeConst  B=inf  A=-inf  init_option=Inherited from block input  x0=0  Ts=-1
  Math Function : Math  Operator=hypot
  Product{,1..3} (4 alike) : Product
  Rate Transition : RateTransition
  Rate Transition1 : RateTransition
  Relay : Relay  OnSwitchValue=0.01  OffSwitchValue=-0.05
  Saturation : Saturate  UpperLimit=1  LowerLimit=-1
  Saturation1 : Saturate  UpperLimit=1  LowerLimit=-1
  Sum : Sum  Inputs=|+-
  Sum1 : Sum  Inputs=|+-
  Sum2 : Sum  Inputs=++|
  Switch : Switch  Criteria=u2 > Threshold  SaturateOnIntegerOverflow=off  InputSameDT=off
  delVd : Outport
  delVq : Outport  Port=2
  Idmax : Outport  Port=3
  Iqmax : Outport  Port=4
  wires:
  Sum/1 -> Gain/1, Relay/1
  Igq/1 -> Rate Transition1/1
  Product1/1 -> Sum2/1
  Gain1/1 -> Product1/2, Product2/1
  Sum1/1 -> Saturation/1
  Product/1 -> Sum1/1
  Product2/1 -> Sum1/2
  Constant/1 -> Sum/2  "IsMaxium"
  Math Function/1 -> Low-Pass Filter/1  "Is"
  [Igq] -> Product3/1, Product2/2
  Switch/1 -> Gain1/1, Product3/2, Product/1
  [Igd] -> Product1/1, Product/2
  Constant2/1 -> Idmax/1
  Constant3/1 -> Iqmax/1
  Gain/1 -> Switch/1
  Constant1/1 -> Switch/3
  Igd/1 -> Rate Transition/1
  Saturation1/1 -> delVq/1
  Relay/1 -> Switch/2
  Saturation/1 -> delVd/1
  Low-Pass Filter/1 -> Sum/1
  Product3/1 -> Sum2/2
  Sum2/1 -> Saturation1/1
  Rate Transition/1 -> Math Function/1, [Igd]
  Rate Transition1/1 -> [Igq], Math Function/2

== system GridFormingConverter/Grid-Forming Converter/Grid-Forming Converter Control/Grid Voltage Reactive Power Support/Modifying Active Power Reference/Computing New Active Power Ref ==
  Iq : Inport
  Vd : Inport  Port=2
  Abs : Abs  SaturateOnIntegerOverflow=off
  Constant : Constant  Value=maxVICurrentLimit*0.96
  Constant1 : Constant  Value=0
  Product : Product
  Sqrt : Sqrt
  Square : Math  Operator=square
  Square1 : Math  Operator=square
  Subtract : Sum  Inputs=-+
  Switch : Switch  Criteria=u2 > Threshold  Threshold=1.15  SaturateOnIntegerOverflow=off  InputSameDT=off
  Pref : Outport
  wires:
  Constant/1 -> Square1/1
  Switch/1 -> Product/2
  Square/1 -> Subtract/1
  Square1/1 -> Subtract/2
  Vd/1 -> Product/1
  Sqrt/1 -> Abs/1
  Iq/1 -> Square/1
  Product/1 -> Pref/1
  Subtract/1 -> Switch/2, Sqrt/1
  Constant1/1 -> Switch/3
  Abs/1 -> Switch/1

== system GridFormingConverter/Grid-Forming Converter/Grid-Forming Converter Control/Grid Voltage Reactive Power Support/Modifying Reactive Power Reference/Changing the Power Reference ==
  Vs : Inport
  Vd : Inport  Port=2
  Pref : Inport  Port=3
  Qref : Inport  Port=4
  Enable : EnablePort
  ActivePowerReference : Subsystem
  Constant1 : Constant  Value=voltreference*0.96
  Estimate Id for Given Iq : Subsystem
  EstimateIqForReactivePower : Subsystem
  Max : MinMax  Function=max  Inputs=2
  ReactivePowerReference : Subsystem
  Prefv : Outport
  Qrefv : Outport  Port=2
  wires:
  EstimateIqForReactivePower/1(Iq) -> Estimate Id for Given Iq/1(Iq), ReactivePowerReference/2(Iq)
  Constant1/1 -> EstimateIqForReactivePower/1(Vmin)
  Vs/1 -> ActivePowerReference/2(Vd), EstimateIqForReactivePower/3(Vs), ReactivePowerReference/1(Vd)
  Estimate Id for Given Iq/1(Id) -> ActivePowerReference/1(Id)
  Pref/1 -> ActivePowerReference/3(Pref)
  ActivePowerReference/1(PrefNew) -> Prefv/1
  ReactivePowerReference/1(QrefNew) -> Max/1
  Max/1 -> Qrefv/1
  Qref/1 -> Max/2
  Vd/1 -> EstimateIqForReactivePower/2(Vd)

== system GridFormingConverter/Grid-Forming Converter/Grid-Forming Converter Control/Grid Voltage Reactive Power Support/Modifying Reactive Power Reference/Hysteresis ==
  Vs : Inport
  AND : Logic  IconShape=distinctive  AllPortsSameDT=off  OutDataTypeStr=boolean
  Compare To Constant : simulink/Logic and Bit Operations/Compare To Constant  relop=<  const=0.9  OutDataTypeStr=boolean
  Compare To Constant1 : simulink/Logic and Bit Operations/Compare To Constant  relop=<  const=0.95  OutDataTypeStr=boolean
  D Latch : simulink_extras/Flip Flops/D Latch
  OR : Logic  Operator=OR  IconShape=distinctive  AllPortsSameDT=off  OutDataTypeStr=boolean
  Terminator : Terminator
  LVFlag : Outport
  wires:
  Compare To Constant1/1 -> AND/1
  D Latch/1 -> AND/2
  AND/1 -> OR/1
  OR/1 -> LVFlag/1
  D Latch/2 -> Terminator/1
  Compare To Constant/1 -> D Latch/1, D Latch/2, OR/2
  Vs/1 -> Compare To Constant1/1, Compare To Constant/1

== system GridFormingConverter/Grid-Forming Converter/Grid-Forming Converter Control/Grid Voltage Reactive Power Support/Modifying Reactive Power Reference/Not Altering the Power Reference ==
  Pref : Inport
  Qref : Inport  Port=2
  Enable : EnablePort
  Prefv : Outport
  Qrefv : Outport  Port=2
  wires:
  Pref/1 -> Prefv/1
  Qref/1 -> Qrefv/1

== system GridFormingConverter/Grid-Forming Converter/Grid-Forming Converter Control/Measurement/Frequency Measurement/Frequency Measurement ==
  abc : Inport
  Constant : Constant
  Discrete-Time Integrator : DiscreteIntegrator  SampleTime=sampleTime  LimitOutput=on  ICPrevOutput=DiscIntNeverNeededParam  ICPrevScaledInput=DiscIntNeverNeededParam
  If : If  IfExpression=u1 > 0.9
  If Action Subsystem : Subsystem  TreatAsAtomicUnit=on
  If Action Subsystem1 : Subsystem  TreatAsAtomicUnit=on
  Merge : Merge
  Postive Sequence : Subsystem
  Freq : Outport
  wires:
  If/1 -> If Action Subsystem/Action
  If/2 -> If Action Subsystem1/Action
  Discrete-Time Integrator/1 -> If Action Subsystem/2(Time), If/1
  abc/1 -> Postive Sequence/1(abc)
  Constant/1 -> Discrete-Time Integrator/1
  If Action Subsystem/1(Freq) -> Merge/1
  If Action Subsystem1/1(Out1) -> Merge/2
  Merge/1 -> Freq/1
  Postive Sequence/1(posSeq) -> If Action Subsystem/1(V)

== system GridFormingConverter/Grid-Forming Converter/Grid-Forming Converter Control/Measurement/abc2dq/Supply Current to dq ==
  abc : Inport
  Angle : Inport  Port=2
  Demux : Demux  Outputs=3
  Park Transform : eeTransforms/Park Transform  AxisAlignment=D-axis  PowerInvariant=off
  Terminator : Terminator
  Igd : Outport  VectorParamsAs1DForOutWhenUnconnected=off
  Igq : Outport  Port=2  VectorParamsAs1DForOutWhenUnconnected=off
  wires:
  Demux/3 -> Terminator/1
  Park Transform/1 -> Demux/1
  Demux/2 -> Igq/1
  Demux/1 -> Igd/1
  abc/1 -> Park Transform/1
  Angle/1 -> Park Transform/2

== system GridFormingConverter/Grid-Forming Converter/Grid-Forming Converter Control/Measurement/abc2dq/Supply Voltage  to dq ==
  Angle : Inport
  abc : Inport  Port=2
  Demux : Demux  Outputs=3
  Park Transform : eeTransforms/Park Transform  AxisAlignment=D-axis  PowerInvariant=off
  Terminator : Terminator
  Vgd : Outport  VectorParamsAs1DForOutWhenUnconnected=off
  Vgq : Outport  Port=2  VectorParamsAs1DForOutWhenUnconnected=off
  wires:
  Demux/3 -> Terminator/1
  Park Transform/1 -> Demux/1
  Demux/2 -> Vgq/1
  Demux/1 -> Vgd/1
  abc/1 -> Park Transform/1
  Angle/1 -> Park Transform/2

== system GridFormingConverter/Grid-Forming Converter/Grid-Forming Converter Control/Power Control/ActivePowerControl/droopControl ==
  Pref : Inport
  Pmeas : Inport  Port=2
  fgrid : Inport  Port=3
  Add : Sum  Inputs=+-
  Constant : Constant
  Constant5 : Constant  Value=pi/2
  Gain : Gain  Gain=powerFreq*2*pi
  Integrator with Wrapped State (Discrete or Continuous) : eeGeneralControl/Integrator with Wrapped State (Discrete or Continuous)  LabelModeActiveChoice=Discrete  WrappedStateUpperValue=2*pi  WrappedStateLowerValue=0  x0=0  Ts=activePowerSampleTime
      settings: LibrarySourceBlock=|
      | ee_sl_lib/General Control/Integrator with
      | Wrapped State
      | (Discrete or Continuous)
  Lead-Lag (Discrete or Continuous) : eeGeneralControl/Lead-Lag (Discrete or Continuous)  T1=droopT1  T2=droopT2  B=inf  A=-inf  init_option=Inherited from block input  x0=0  Ts=activePowerSampleTime
      settings: LibrarySourceBlock=|
      | ee_sl_lib/General Control/Lead-Lag
      | (Discrete or Continuous)
  Low-Pass Filter (Discrete or Continuous) : eeGeneralControl/Low-Pass Filter (Discrete or Continuous)  K=1  T=droopTC  B=inf  A=-inf  init_option=Specify as parameter  x0=0  Ts=activePowerSampleTime
  Sum : Sum  Inputs=|-+
  Sum1 : Sum  Inputs=|-+
  Terminator : Terminator
  mp : Gain  Gain=droopSlope
  Theta : Outport
  w : Outport  Port=2
  wires:
  Low-Pass Filter (Discrete or Continuous)/1 -> Sum1/1
  mp/1 -> Low-Pass Filter (Discrete or Continuous)/1
  Sum/1 -> mp/1
  Pmeas/1 -> Lead-Lag (Discrete or Continuous)/1
  Add/1 -> Theta/1
  Constant5/1 -> Add/2
  Pref/1 -> Sum/1
  Gain/1 -> Integrator with Wrapped State (Discrete or Continuous)/1, w/1
  Lead-Lag (Discrete or Continuous)/1 -> Sum/2
  Integrator with Wrapped State (Discrete or Continuous)/1 -> Add/1
  Constant/1 -> Sum1/2
  Sum1/1 -> Gain/1
  fgrid/1 -> Terminator/1

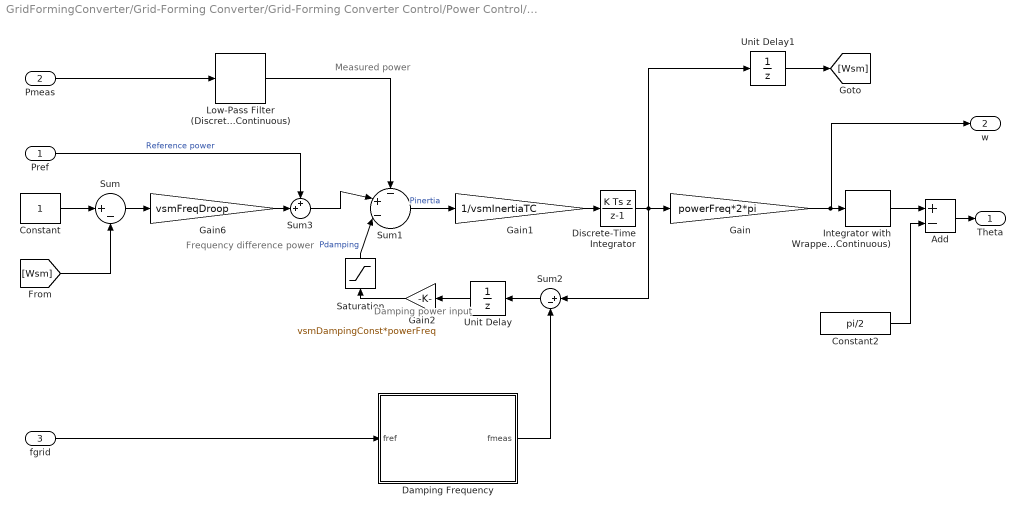
== system GridFormingConverter/Grid-Forming Converter/Grid-Forming Converter Control/Power Control/ActivePowerControl/vsmControl ==
  note: Measured power
  note: Frequency difference power
  note: Damping power input
  Pref : Inport
  Pmeas : Inport  Port=2
  fgrid : Inport  Port=3
  Add : Sum  Inputs=+-
  Constant : Constant
  Constant2 : Constant  Value=pi/2
  Damping Frequency : Subsystem  Variant=on  VariantControlMode=label  VariantControl=Choice  LabelModeActiveChoice=freqMeas
  Discrete-Time Integrator : DiscreteIntegrator  IntegratorMethod=Integration: Backward Euler  InitialCondition=1  SampleTime=activePowerSampleTime  LimitOutput=on  UpperSaturationLimit=1.1  LowerSaturationLimit=0.9  ICPrevOutput=DiscIntNeverNeededParam  ICPrevScaledInput=DiscIntNeverNeededParam
  Gain : Gain  Gain=powerFreq*2*pi
  Gain1 : Gain  Gain=1/vsmInertiaTC
  Gain2 : Gain  Gain=vsmDampingConst*powerFreq
  Gain6 : Gain  Gain=vsmFreqDroop
  Integrator with Wrapped State (Discrete or Continuous) : eeGeneralControl/Integrator with Wrapped State (Discrete or Continuous)  LabelModeActiveChoice=Discrete  WrappedStateUpperValue=2*pi  WrappedStateLowerValue=0  x0=0  Ts=activePowerSampleTime
      settings: LibrarySourceBlock=|
      | ee_sl_lib/General Control/Integrator with
      | Wrapped State
      | (Discrete or Continuous)
  Low-Pass Filter (Discrete or Continuous) : eeGeneralControl/Low-Pass Filter (Discrete or Continuous)  K=1  T=vsmPmeasFilterTC  B=inf  A=-inf  init_option=Specify as parameter  x0=0  Ts=activePowerSampleTime
  Saturation : Saturate  UpperLimit=dampingPowerMaxLimit  LowerLimit=dampingPowerMinLimit
  Sum : Sum  Inputs=|+-
  Sum1 : Sum  Inputs=-+-|
  Sum2 : Sum  Inputs=|+-
  Sum3 : Sum  Inputs=++|
  Unit Delay : UnitDelay  SampleTime=-1  HasFrameUpgradeWarning=on
  Unit Delay1 : UnitDelay  SampleTime=-1  HasFrameUpgradeWarning=on
  Theta : Outport
  w : Outport  Port=2
  wires:
  Integrator with Wrapped State (Discrete or Continuous)/1 -> Add/1
  Sum1/1 -> Gain1/1  "Pinertia"
  Sum/1 -> Gain6/1
  Constant2/1 -> Add/2
  Add/1 -> Theta/1
  Pmeas/1 -> Low-Pass Filter (Discrete or Continuous)/1
  Discrete-Time Integrator/1 -> Gain/1, Unit Delay1/1, Sum2/1
  [Wsm] -> Sum/2
  Low-Pass Filter (Discrete or Continuous)/1 -> Sum1/1
  Pref/1 -> Sum3/1  "Reference power"
  Gain2/1 -> Saturation/1
  Sum3/1 -> Sum1/2
  Sum2/1 -> Unit Delay/1
  Gain1/1 -> Discrete-Time Integrator/1
  Gain/1 -> Integrator with Wrapped State (Discrete or Continuous)/1, w/1
  Unit Delay/1 -> Gain2/1
  Constant/1 -> Sum/1
  Unit Delay1/1 -> [Wsm]
  Saturation/1 -> Sum1/3  "Pdamping"
  Gain6/1 -> Sum3/2
  fgrid/1 -> Damping Frequency/1(fref)
  Damping Frequency/1(fmeas) -> Sum2/2

== system GridFormingConverter/Grid-Forming Converter/Grid-Forming Converter Control/VoltageCurrentControl/Controller/Id Current Limiting ==
  Imax : Inport
  Id : Inport  Port=2
  Abs : Abs  SaturateOnIntegerOverflow=off
  Rate Transition : RateTransition
  Switch : Switch  Criteria=u2 > Threshold  SaturateOnIntegerOverflow=off  InputSameDT=off
  Idref : Outport
  wires:
  Id/1 -> Rate Transition/1
  Abs/1 -> Switch/2
  Imax/1 -> Abs/1, Switch/1
  Switch/1 -> Idref/1
  Rate Transition/1 -> Switch/3

== system GridFormingConverter/Grid-Forming Converter/Grid-Forming Converter Control/VoltageCurrentControl/Controller/Iq Current Limiting ==
  Imax : Inport
  Iq : Inport  Port=2
  Abs : Abs  SaturateOnIntegerOverflow=off
  Switch : Switch  Criteria=u2 > Threshold  SaturateOnIntegerOverflow=off  InputSameDT=off
  Iqref : Outport
  wires:
  Iq/1 -> Switch/3
  Abs/1 -> Switch/2
  Imax/1 -> Abs/1, Switch/1
  Switch/1 -> Iqref/1

== system GridFormingConverter/Grid-Forming Converter/Grid-Forming Converter Control/VoltageCurrentControl/Controller/Voltage control ==
  e : Inport
  Discrete-Time Integrator : DiscreteIntegrator  IntegratorMethod=Integration: Backward Euler  SampleTime=voltControlTs  LimitOutput=on  UpperSaturationLimit=VdMaxCt  LowerSaturationLimit=VdMinCt  ICPrevOutput=DiscIntNeverNeededParam  ICPrevScaledInput=DiscIntNeverNeededParam
  Ki : Gain  Gain=VdIGain
  Kp : Gain  Gain=vdPGain
  Limit : Saturate  UpperLimit=VdMaxCt  LowerLimit=VdMinCt
  Sum7 : Sum  Inputs=|++
  u : Outport  VectorParamsAs1DForOutWhenUnconnected=off
  wires:
  Discrete-Time Integrator/1 -> Sum7/2
  Kp/1 -> Sum7/1
  Limit/1 -> u/1
  Ki/1 -> Discrete-Time Integrator/1
  Sum7/1 -> Limit/1
  e/1 -> Kp/1, Ki/1

== system GridFormingConverter/Grid-Forming Converter/Grid-Forming Converter Control/VoltageCurrentControl/Controller/Voltage control1 ==
  e : Inport
  Discrete-Time Integrator : DiscreteIntegrator  IntegratorMethod=Integration: Backward Euler  SampleTime=voltControlTs  LimitOutput=on  UpperSaturationLimit=VqMaxCt  LowerSaturationLimit=VqMinCt  ICPrevOutput=DiscIntNeverNeededParam  ICPrevScaledInput=DiscIntNeverNeededParam
  Ki : Gain  Gain=VqIGain
  Kp : Gain  Gain=VqPGain
  Limit : Saturate  UpperLimit=VqMaxCt  LowerLimit=VqMinCt
  Sum7 : Sum  Inputs=|++
  u : Outport  VectorParamsAs1DForOutWhenUnconnected=off
  wires:
  Discrete-Time Integrator/1 -> Sum7/2
  Sum7/1 -> Limit/1
  e/1 -> Ki/1, Kp/1
  Kp/1 -> Sum7/1
  Ki/1 -> Discrete-Time Integrator/1
  Limit/1 -> u/1

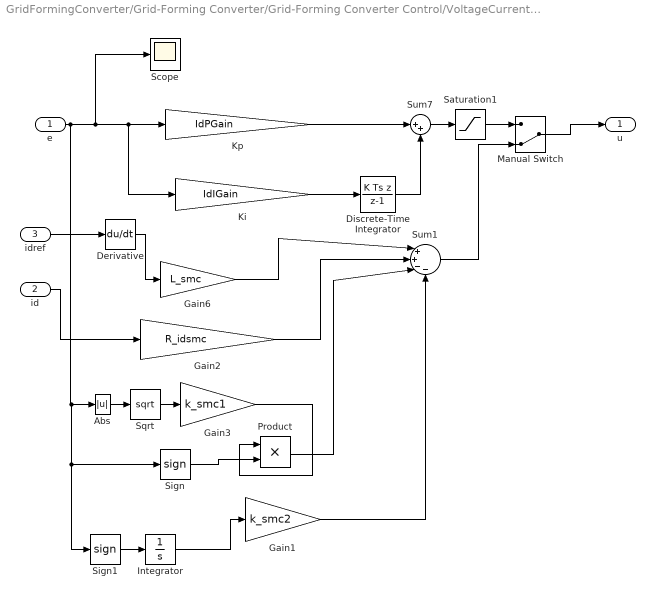
== system GridFormingConverter/Grid-Forming Converter/Grid-Forming Converter Control/VoltageCurrentControl/Controller/d-axis current control ==
  e : Inport
  id : Inport  Port=2
  idref : Inport  Port=3
  Abs : Abs  SaturateOnIntegerOverflow=off
  Derivative : Derivative
  Discrete-Time Integrator : DiscreteIntegrator  IntegratorMethod=Integration: Backward Euler  SampleTime=currentControlTs  LimitOutput=on  UpperSaturationLimit=4  LowerSaturationLimit=-4  ICPrevOutput=DiscIntNeverNeededParam  ICPrevScaledInput=DiscIntNeverNeededParam
  Gain1 : Gain  Gain=k_smc2
  Gain2 : Gain  Gain=R_idsmc
  Gain3 : Gain  Gain=k_smc1
  Gain6 : Gain  Gain=L_smc
  Integrator : Integrator
  Ki : Gain  Gain=IdIGain
  Kp : Gain  Gain=IdPGain
  Manual Switch : ManualSwitch  CurrentSetting=0
  Product : Product
  Saturation1 : Saturate  UpperLimit=4  LowerLimit=-4
  Scope : Scope
      settings: ActiveDisplayYMinimum=-0.22577611192495703  ActiveDisplayYMaximum=0.41180956799166185
  Sign : Signum
  Sign1 : Signum
  Sqrt : Sqrt
  Sum1 : Sum  Inputs=|++--
  Sum7 : Sum  Inputs=|++
  u : Outport  VectorParamsAs1DForOutWhenUnconnected=off
  wires:
  Discrete-Time Integrator/1 -> Sum7/2
  e/1 -> Scope/1, Ki/1, Kp/1, Sign/1, Sign1/1, Abs/1
  Kp/1 -> Sum7/1
  Ki/1 -> Discrete-Time Integrator/1
  Manual Switch/1 -> u/1
  Sum7/1 -> Saturation1/1
  id/1 -> Gain2/1
  Derivative/1 -> Gain6/1
  Gain2/1 -> Sum1/2
  Gain3/1 -> Product/1
  Saturation1/1 -> Manual Switch/1
  Product/1 -> Sum1/3
  idref/1 -> Derivative/1
  Gain6/1 -> Sum1/1
  Sum1/1 -> Manual Switch/2
  Sqrt/1 -> Gain3/1
  Sign/1 -> Product/2
  Sign1/1 -> Integrator/1
  Integrator/1 -> Gain1/1
  Gain1/1 -> Sum1/4
  Abs/1 -> Sqrt/1

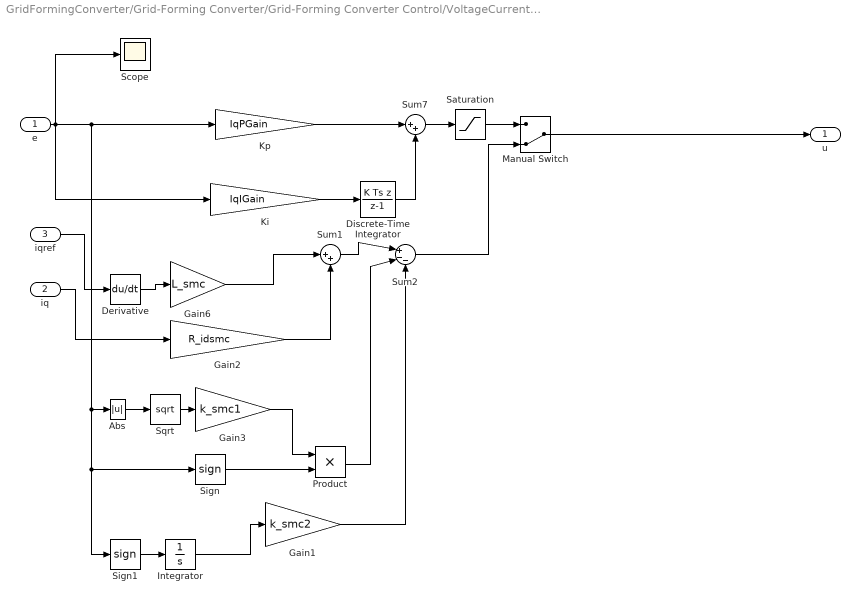
== system GridFormingConverter/Grid-Forming Converter/Grid-Forming Converter Control/VoltageCurrentControl/Controller/q-axis current control ==
  e : Inport
  iq : Inport  Port=2
  iqref : Inport  Port=3
  Abs : Abs  SaturateOnIntegerOverflow=off
  Derivative : Derivative
  Discrete-Time Integrator : DiscreteIntegrator  IntegratorMethod=Integration: Backward Euler  SampleTime=currentControlTs  LimitOutput=on  UpperSaturationLimit=3  LowerSaturationLimit=-3  ICPrevOutput=DiscIntNeverNeededParam  ICPrevScaledInput=DiscIntNeverNeededParam
  Gain1 : Gain  Gain=k_smc2
  Gain2 : Gain  Gain=R_idsmc
  Gain3 : Gain  Gain=k_smc1
  Gain6 : Gain  Gain=L_smc
  Integrator : Integrator
  Ki : Gain  Gain=IqIGain
  Kp : Gain  Gain=IqPGain
  Manual Switch : ManualSwitch  CurrentSetting=0
  Product : Product
  Saturation : Saturate  UpperLimit=3  LowerLimit=-3
  Scope : Scope
      settings: ActiveDisplayYMinimum=-0.24012972531706872  ActiveDisplayYMaximum=0.22900536028160953  DataLoggingVariableName=ScopeData2
  Sign : Signum
  Sign1 : Signum
  Sqrt : Sqrt
  Sum1 : Sum  Inputs=|++
  Sum2 : Sum  Inputs=|+--
  Sum7 : Sum  Inputs=|++
  u : Outport  VectorParamsAs1DForOutWhenUnconnected=off
  wires:
  Ki/1 -> Discrete-Time Integrator/1
  Kp/1 -> Sum7/1
  Discrete-Time Integrator/1 -> Sum7/2
  Manual Switch/1 -> u/1
  Sum7/1 -> Saturation/1
  Saturation/1 -> Manual Switch/1
  iqref/1 -> Derivative/1
  Gain6/1 -> Sum1/1
  Gain2/1 -> Sum1/2
  Derivative/1 -> Gain6/1
  Sum1/1 -> Sum2/1
  iq/1 -> Gain2/1
  Sum2/1 -> Manual Switch/2
  Sign/1 -> Product/2
  Product/1 -> Sum2/2
  e/1 -> Sign/1, Sign1/1, Abs/1, Kp/1, Ki/1, Scope/1
  Sign1/1 -> Integrator/1
  Gain1/1 -> Sum2/3
  Integrator/1 -> Gain1/1
  Sqrt/1 -> Gain3/1
  Gain3/1 -> Product/1
  Abs/1 -> Sqrt/1
